simulink model "chp71"  (R2019a)
settings: Solver=VariableStepAuto  StartTime=0.0  StopTime=10.0  RelTol=1e-3
settings Model: Creator=zkibria  LastModifiedBy=zkibria

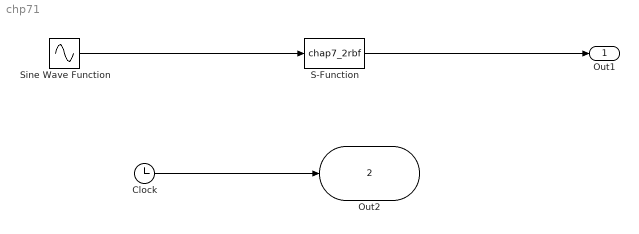
== system chp71 ==
  Clock : Clock
  S-Function : S-Function  FunctionName=chap7_2rbf  SFunctionDeploymentMode=off  EnableBusSupport=off
  Sine Wave Function : Sin  SampleTime=0
  Out1 : Outport  SignalName=y
  Out2 : Outport  Port=2  SignalName=t
  wires:
  Clock/1 -> Out2/1
  Sine Wave Function/1 -> S-Function/1
  S-Function/1 -> Out1/1
